simulink model "part03"  (R2022a)
settings: Solver=VariableStepAuto  StartTime=0.0  StopTime=100  RelTol=1e-3
settings Model: Creator=ac133867  LastModifiedBy=cunis
settings DebuggingCC: UnconnectedInputMsg=warning  UnconnectedOutputMsg=warning  UnconnectedLineMsg=warning
settings RTWCC: DLArmComputeVersion=19.05

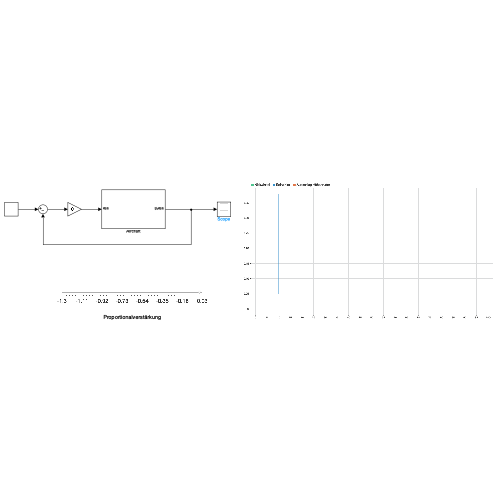
[thumbnail: Simulink's stored preview of the top-level diagram]
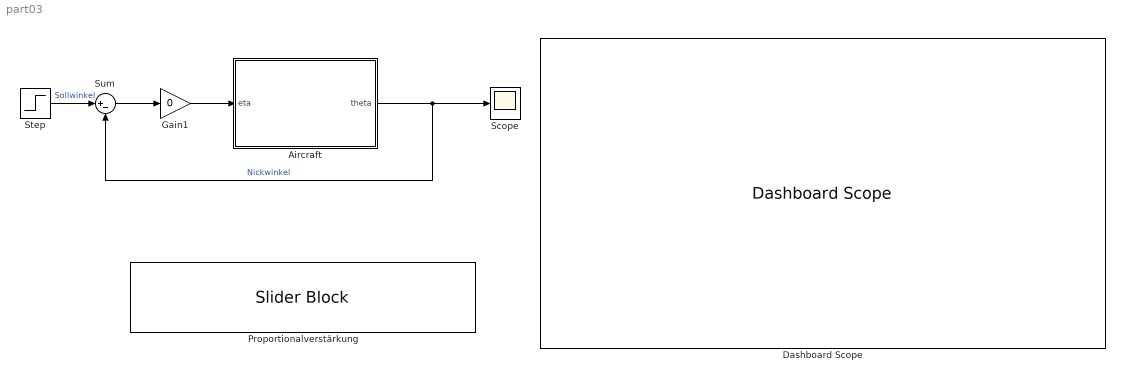
== system part03 ==
  Aircraft : Subsystem
  Dashboard Scope : DashboardScope
  Gain1 : Gain  Gain=0
  Proportionalverstärkung : SliderBlock  LabelPosition=Hide  ScaleMin=-1.3  ScaleMax=0.03
  Scope : Scope
  Step : Step  Time=10  Before=0.049807151144250  After=0.38  SampleTime=0
  Sum : Sum  Inputs=|+-
  wires:
  Step/1 -> Sum/1  "Sollwinkel"
  Sum/1 -> Gain1/1
  Aircraft/1(theta) -> Scope/1, Sum/2  "Nickwinkel"
  Gain1/1 -> Aircraft/1(eta)

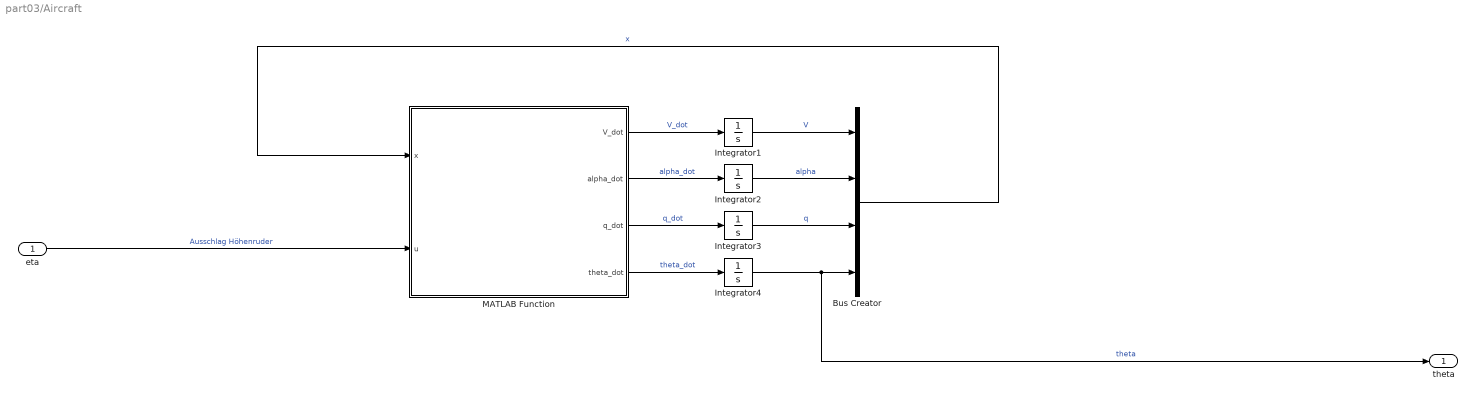
== system part03/Aircraft ==
  eta : Inport
  Bus Creator : BusCreator  Inputs=4
  Integrator1 : Integrator  InitialCondition=44.872852763976020
  Integrator2 : Integrator  InitialCondition=0.049300445857312
  Integrator3 : Integrator
  Integrator4 : Integrator  InitialCondition=0.049807151144250
  MATLAB Function : MATLAB Function  TreatAsAtomicUnit=on
  theta : Outport
  wires:
  Integrator3/1 -> Bus Creator/3  "q"
  MATLAB Function/2(alpha_dot) -> Integrator2/1  "alpha_dot"
  Integrator4/1 -> theta/1, Bus Creator/4  "theta"
  Bus Creator/1 -> MATLAB Function/1(x)  "x"
  MATLAB Function/1(V_dot) -> Integrator1/1  "V_dot"
  Integrator1/1 -> Bus Creator/1  "V"
  MATLAB Function/4(theta_dot) -> Integrator4/1  "theta_dot"
  Integrator2/1 -> Bus Creator/2  "alpha"
  eta/1 -> MATLAB Function/2(u)  "Ausschlag Höhenruder"
  MATLAB Function/3(q_dot) -> Integrator3/1  "q_dot"

== matlab function part03/Aircraft/MATLAB Function ==
  data: x input size=[4 1]; u input; V_dot output; alpha_dot output; q_dot output; theta_dot output
function [V_dot, alpha_dot, q_dot, theta_dot]= poly_long_dyn(x,u)



% fixed trim values
delta0  = 14.33;   % percent
            


eta_trim = 0.048920000000000;

X = [x(1); x(2); x(3); x(4)];
U = [u + eta_trim; delta0];



%% Polynomial Dynamics
f1 = @(V,alpha,q,theta,eta,F) +1.233e-8*V.^4.*q.^2         + 4.853e-9.*alpha.^3.*F.^3    + 3.705e-5*V.^3.*alpha.*q      ...
                             - 2.184e-6*V.^3.*q.^2         + 2.203e-2*V.^2.*alpha.^3     - 2.836e-6*alpha.^3.*F.^2      ...
                             + 3.885e-7*alpha.^2.*F.^3     - 1.069e-6*V.^3.*q            - 4.517e-2*V.^2.*alpha.^2      ...
                             - 2.140e-3*V.^2.*alpha.*eta   - 3.282e-3*V.^2.*alpha.*q     - 8.901e-4*V.^2.*eta.^2        ...
                             + 9.677e-5*V.^2.*q.^2         - 2.037e-4*alpha.^3.*F        - 2.270e-4*alpha.^2.*F.^2      ...
                             - 2.912e-8*alpha.*F.^3        + 1.591e-3*V.^2.*alpha        - 4.077e-4*V.^2.*eta           ...
                             + 9.475e-5*V.^2.*q            - 1.637   *alpha.^3           - 1.631e-2*alpha.^2.*F         ...
                             + 4.903   *alpha.^2.*theta    - 4.903   *alpha.*theta.^2    + 1.702e-5*alpha.*F.^2         ...
                             - 7.771e-7*F.^3               + 1.634   *theta.^3           - 4.319e-4*V.^2                ...
                             - 2.142e-1*alpha.^2           + 1.222e-3*alpha.*F           + 4.541e-4*F.^2                ...
                             + 9.823   *alpha              + 3.261e-2*F                  - 9.807.*theta      + 4.284e-1;

                      
% change of angle of attack
f2 = @(V,alpha,q,theta,eta,F) -3.709e-11*V.^5.*   q.^2     + 6.869e-11*V.*alpha.^3.*F.^3 + 7.957e-10*V.^4.*alpha.*q     ...
                             + 9.860e-9 *V.^4.*   q.^2     + 1.694e-5 *V.^3.*alpha.^3    - 4.015e-8 *V.*alpha.^3.*F.^2  ...
                             - 7.722e-12*V.*alpha.^2.*F.^3 - 6.086e-9 *alpha.^3.*F.^3    - 2.013e-8 *V.^4.*q            ...
                             - 5.180e-5 *V.^3.*alpha.^2    - 2.720e-6 *V.^3.*alpha.*eta  - 1.410e-7 *V.^3.*alpha.*q     ...
                             + 7.352e-7 *V.^3.*eta.^2      - 8.736e-7 *V.^3.*q.^2        - 1.501e-3 *V.^2.*alpha.^3     ...
                             - 2.883e-6 *V.*alpha.^3.*F    + 4.513e-9 *V.*alpha.^2.*F.^2 - 4.121e-10*V.*alpha.*F.^3     ...
                             + 3.557e-6 *alpha.^3.*F.^2    + 6.841e-10*alpha.^2.*F.^3    + 4.151e-5 *V.^3.*alpha        ...
                             + 3.648e-6 *V.^3.*eta         + 3.566e-6 *V.^3.*q           + 6.246e-6 *V.^2.*alpha.*q     ...
                             + 4.589e-3 *V.^2.*alpha.^2                                  - 6.514e-5 *V.^2.*eta.^2       ...
                             + 2.580e-5 *V.^2.*q.^2        - 3.787e-5 *V.*alpha.^3       + 3.241e-7 *V.*alpha.^2.*F     ...
                             + 2.409e-7 *V.*alpha.*F.^2    + 1.544e-11*V.*F.^3           + 2.554e-4 *alpha.^3.*F        ...
                             - 3.998e-7 *alpha.^2.*F.^2    + 3.651e-8 *alpha.*F.^3       + 4.716e-7 *V.^3               ...
                             - 3.677e-3 *V.^2*alpha        - 3.231e-4 *V.^2.*eta         - 1.579e-4 *V.^2.*q            ...
                             + 2.605e-3 *V.*alpha.^2       + 1.730e-5 *V.*alpha.*F       - 5.201e-3 *V.*alpha.*theta    ...
                             - 9.026e-9 *V.*F.^2           + 2.601e-3 *V.*theta.^2       + 3.355e-3 *alpha.^3           ...
                             - 2.872e-5 *alpha.^2.*F       - 2.134e-5 *alpha.*F.^2       - 1.368e-9 *F.^3               ...
                             - 4.178e-5 *V.^2              + 2.272e-4 *V.*alpha          - 6.483e-7 *V.*F               ...
                             - 2.308e-1 *alpha.^2          - 1.532e-3 *alpha.*F          + 4.608e-1 *alpha.*theta       ...
                             - 2.304e-1 *theta.^2          + 7.997e-7 *F.^2              - 5.210e-3 *V                  ...
                             - 2.013e-2 *alpha             + 5.744e-5 *F          + q    + 4.616e-1;
                         
% change of pitch rate                         
f3 = @(V,alpha,q,theta,eta,F) -6.573e-9*V.^5.*    q.^3     + 1.747e-6*V.^4.*q.^3         - 1.548e-4*V.^3.*q.^3          ...
                             - 3.569e-3*V.^2.*alpha.^3     + 4.571e-3*V.^2.*q.^3         + 4.953e-5*V.^3.*q             ...
                             + 9.596e-3*V.^2.*alpha.^2     + 2.049e-2*V.^2.*alpha.*eta   - 2.431e-2*V.^2.*alpha         ...
                             - 3.063e-2*V.^2.*eta          - 4.388e-3*V.^2.*q            - 2.594e-7*F.^3                ...
                             + 2.461e-3*V.^2               + 1.516e-4*F.^2               + 1.089e-2*F        + 1.430e-1;                         

% change of pitch angle
f4 = @(V,alpha,q,theta,eta,F)  q;



V_dot     = f1(X(1,:),X(2,:),X(3,:),X(4,:),U(1,:),U(2,:));
alpha_dot = f2(X(1,:),X(2,:),X(3,:),X(4,:),U(1,:),U(2,:));

q_dot     = f3(X(1,:),X(2,:),X(3,:),X(4,:),U(1,:),U(2,:));
theta_dot = f4(X(1,:),X(2,:),X(3,:),X(4,:),U(1,:),U(2,:));
